simulink model "Instalatie_cu_filtru"  (R2024b)
settings: Solver=VariableStepAuto  StartTime=0.0  StopTime=1000  RelTol=1e-3  EnableMultiTasking=on
values from neighbouring files (symbols this model uses):
  k = 0.046    [Coeficienti.m]
  k11 = k2^2 + 4* (k - k3) * k1    (= 0.1165386)    [Coeficienti.m]
  k12 = 8* (k - k3)    (= 0.3728)    [Coeficienti.m]
  k13 = 2* (k - k3)    (= 0.0932)    [Coeficienti.m]
  k2 = -0.015    [Coeficienti.m]
  keta = 8e-5    (= 8e-05)    [Coeficienti.m]
  u0 = 6.6    [Coeficienti.m]
settings Model: Creator=otudo  LastModifiedBy=receaalex
settings SolverCC: AlgebraicLoopSolver=TrustRegion
settings DataIOCC: ReturnWorkspaceOutputs=off
settings OptimizationCC: LifeSpan=inf
settings DebuggingCC: UnconnectedInputMsg=warning  UnconnectedOutputMsg=warning  UnconnectedLineMsg=warning  SFUnexpectedBacktrackingDiag=warning  SFNoUnconditionalDefaultTransitionDiag=warning  ArithmeticOperatorsInVariantConditions=warning
settings ModelReferenceCC: EnableRefExpFcnMdlSchedulingChecks=on
settings SFSimCC: SimUseLocalCustomCode=off  CustomCodeUndefinedFunction=UseInterfaceOnly
settings RTWCC: RTWUseLocalCustomCode=off  GPUComputeCapability=3.5
settings CodeAppCC: StateflowObjectComments=on
settings GRTTargetCC: TargetLangStandard=C89/C90 (ANSI)
settings ConfigComp: CovMetricSettings=dw  CovSaveCumulativeToWorkspaceVar=on  CovSaveSingleToWorkspaceVar=on  CovExternalEMLEnable=off

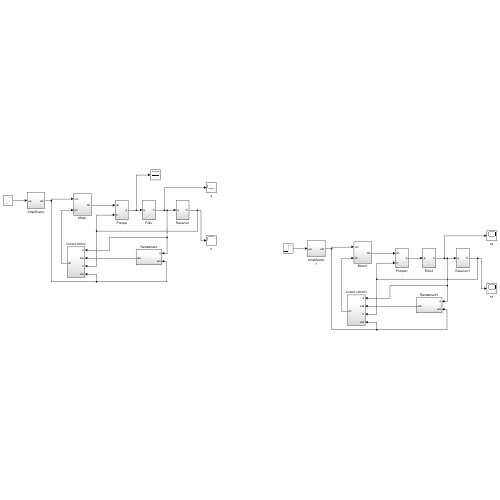
[thumbnail: Simulink's stored preview of the top-level diagram]
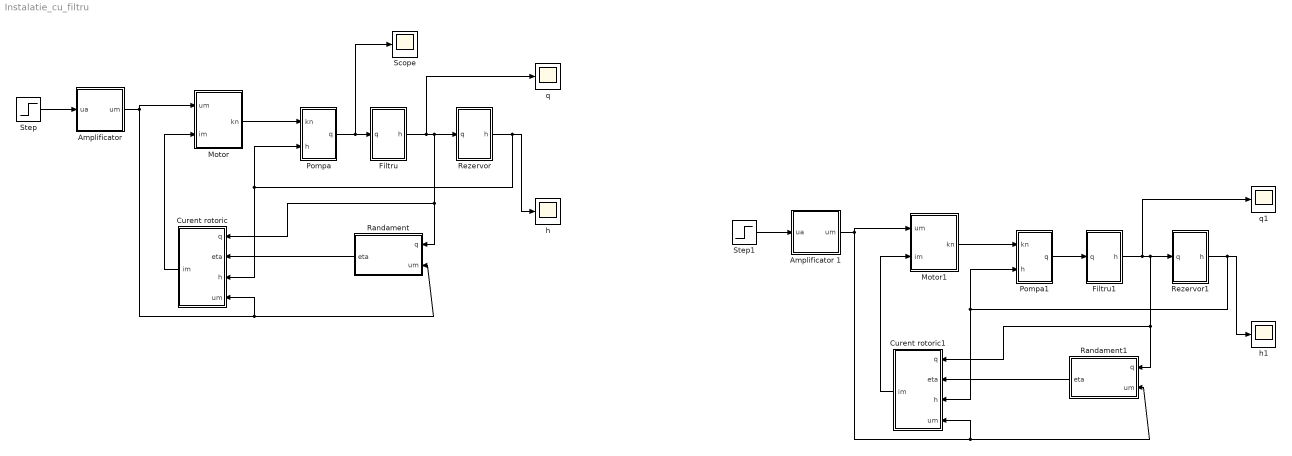
== system Instalatie_cu_filtru ==
  "Amplificator " : Subsystem
  Amplificator 1 : Subsystem
  Curent rotoric : Subsystem
  Curent rotoric1 : Subsystem
  Filtru : Subsystem
  Filtru1 : Subsystem
  Motor : Subsystem
  Motor1 : Subsystem
  Pompa : Subsystem
  Pompa1 : Subsystem
  Randament : Subsystem
  Randament1 : Subsystem
  Rezervor : Subsystem
  Rezervor1 : Subsystem
  Scope : Scope
  Step : Step  Before=u0  After=u0+0.5  SampleTime=0
  Step1 : Step  After=u0  SampleTime=0
  h : Scope
  h1 : Scope
  q : Scope
  q1 : Scope
  wires:
  Filtru/1(h) -> q/1, Curent rotoric/1(q), Randament/1(q), Rezervor/1(q)
  Step/1 -> "Amplificator "/1(ua)
  Randament/1(eta) -> Curent rotoric/2(eta)
  Rezervor/1(h) -> Curent rotoric/3(h), Pompa/2(h), h/1
  Pompa/1(q) -> Scope/1, Filtru/1(q)
  Curent rotoric/1(im) -> Motor/2(im)
  "Amplificator "/1(um) -> Curent rotoric/4(um), Randament/2(um), Motor/1(um)
  Motor/1(kn) -> Pompa/1(kn)
  Pompa1/1(q) -> Filtru1/1(q)
  Motor1/1(kn) -> Pompa1/1(kn)
  Step1/1 -> Amplificator 1/1(ua)
  Rezervor1/1(h) -> Curent rotoric1/3(h), Pompa1/2(h), h1/1
  Randament1/1(eta) -> Curent rotoric1/2(eta)
  Amplificator 1/1(um) -> Curent rotoric1/4(um), Randament1/2(um), Motor1/1(um)
  Curent rotoric1/1(im) -> Motor1/2(im)
  Filtru1/1(h) -> q1/1, Curent rotoric1/1(q), Randament1/1(q), Rezervor1/1(q)

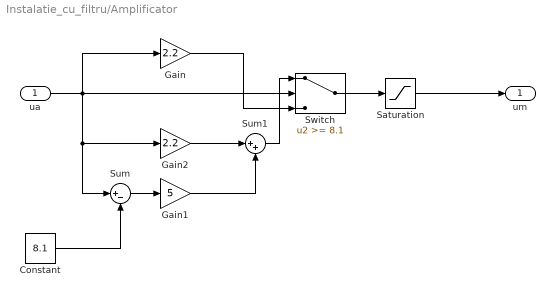
== system Instalatie_cu_filtru/Amplificator  ==
  ua : Inport
  Constant : Constant  Value=8.1
  Gain : Gain  Gain=2.2
  Gain1 : Gain  Gain=5
  Gain2 : Gain  Gain=2.2
  Saturation : Saturate  UpperLimit=22  LowerLimit=0
  Sum : Sum  Inputs=|+-
  Sum1 : Sum  Inputs=|++
  Switch : Switch  Threshold=8.1  SaturateOnIntegerOverflow=off  InputSameDT=off
  um : Outport
  wires:
  Gain/1 -> Switch/3
  Gain1/1 -> Sum1/2
  Switch/1 -> Saturation/1
  Constant/1 -> Sum/2
  Gain2/1 -> Sum1/1
  Sum/1 -> Gain1/1
  Saturation/1 -> um/1
  ua/1 -> Sum/1, Gain2/1, Gain/1, Switch/2
  Sum1/1 -> Switch/1

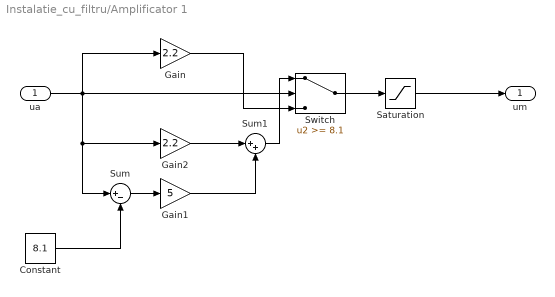
== system Instalatie_cu_filtru/Amplificator 1 ==
  ua : Inport
  Constant : Constant  Value=8.1
  Gain : Gain  Gain=2.2
  Gain1 : Gain  Gain=5
  Gain2 : Gain  Gain=2.2
  Saturation : Saturate  UpperLimit=22  LowerLimit=0
  Sum : Sum  Inputs=|+-
  Sum1 : Sum  Inputs=|++
  Switch : Switch  Threshold=8.1  SaturateOnIntegerOverflow=off  InputSameDT=off
  um : Outport
  wires:
  Gain/1 -> Switch/3
  Gain1/1 -> Sum1/2
  Switch/1 -> Saturation/1
  Constant/1 -> Sum/2
  Gain2/1 -> Sum1/1
  Sum/1 -> Gain1/1
  Saturation/1 -> um/1
  ua/1 -> Sum/1, Gain2/1, Gain/1, Switch/2
  Sum1/1 -> Switch/1

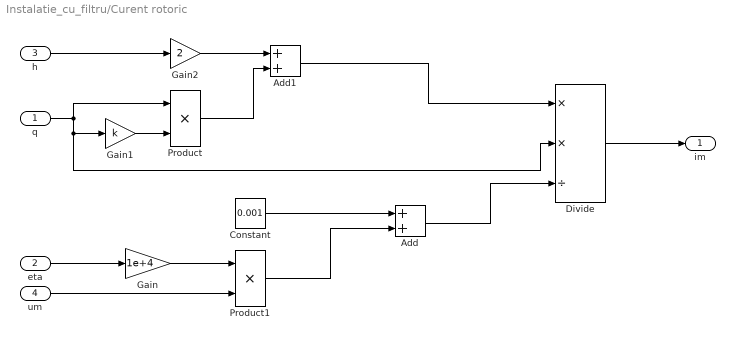
== system Instalatie_cu_filtru/Curent rotoric ==
  q : Inport
  eta : Inport  Port=2
  h : Inport  Port=3
  um : Inport  Port=4
  Add : Sum
  Add1 : Sum
  Constant : Constant  Value=0.001
  Divide : Product  Inputs=**/
  Gain : Gain  Gain=1e+4
  Gain1 : Gain  Gain=k
  Gain2 : Gain  Gain=2
  Product : Product
  Product1 : Product
  im : Outport
  wires:
  Add1/1 -> Divide/1
  Constant/1 -> Add/1
  Add/1 -> Divide/3
  Gain1/1 -> Product/2
  Product/1 -> Add1/2
  um/1 -> Product1/2
  Product1/1 -> Add/2
  Divide/1 -> im/1
  Gain/1 -> Product1/1
  Gain2/1 -> Add1/1
  eta/1 -> Gain/1
  q/1 -> Divide/2, Gain1/1, Product/1
  h/1 -> Gain2/1

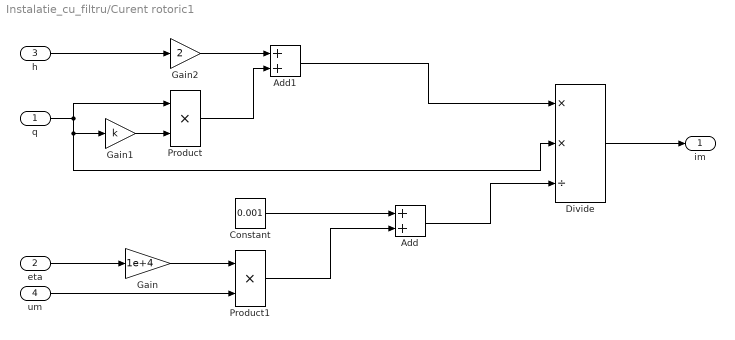
== system Instalatie_cu_filtru/Curent rotoric1 ==
  q : Inport
  eta : Inport  Port=2
  h : Inport  Port=3
  um : Inport  Port=4
  Add : Sum
  Add1 : Sum
  Constant : Constant  Value=0.001
  Divide : Product  Inputs=**/
  Gain : Gain  Gain=1e+4
  Gain1 : Gain  Gain=k
  Gain2 : Gain  Gain=2
  Product : Product
  Product1 : Product
  im : Outport
  wires:
  Add1/1 -> Divide/1
  Constant/1 -> Add/1
  Add/1 -> Divide/3
  Gain1/1 -> Product/2
  Product/1 -> Add1/2
  um/1 -> Product1/2
  Product1/1 -> Add/2
  Divide/1 -> im/1
  Gain/1 -> Product1/1
  Gain2/1 -> Add1/1
  eta/1 -> Gain/1
  q/1 -> Divide/2, Gain1/1, Product/1
  h/1 -> Gain2/1

== system Instalatie_cu_filtru/Filtru ==
  q : Inport
  Integrator : Integrator  InitialCondition=36.6
  Sum : Sum  Inputs=|+-
  h : Outport
  wires:
  Sum/1 -> Integrator/1
  q/1 -> Sum/1
  Integrator/1 -> h/1, Sum/2

== system Instalatie_cu_filtru/Filtru1 ==
  q : Inport
  Integrator : Integrator
  Sum : Sum  Inputs=|+-
  h : Outport
  wires:
  Sum/1 -> Integrator/1
  q/1 -> Sum/1
  Integrator/1 -> h/1, Sum/2

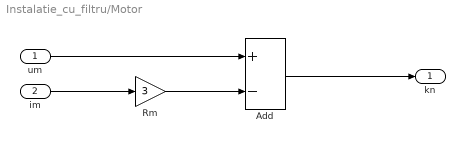
== system Instalatie_cu_filtru/Motor ==
  um : Inport
  im : Inport  Port=2
  Add : Sum  Inputs=+-
  "Rm " : Gain  Gain=3
  kn : Outport
  wires:
  "Rm "/1 -> Add/2
  Add/1 -> kn/1
  um/1 -> Add/1
  im/1 -> "Rm "/1

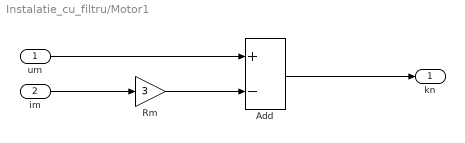
== system Instalatie_cu_filtru/Motor1 ==
  um : Inport
  im : Inport  Port=2
  Add : Sum  Inputs=+-
  "Rm " : Gain  Gain=3
  kn : Outport
  wires:
  "Rm "/1 -> Add/2
  Add/1 -> kn/1
  um/1 -> Add/1
  im/1 -> "Rm "/1

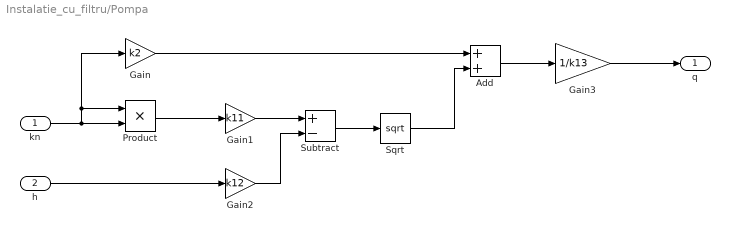
== system Instalatie_cu_filtru/Pompa ==
  kn : Inport
  h : Inport  Port=2
  Add : Sum
  Gain : Gain  Gain=k2
  Gain1 : Gain  Gain=k11
  Gain2 : Gain  Gain=k12
  Gain3 : Gain  Gain=1/k13
  Product : Product
  Sqrt : Sqrt
  Subtract : Sum  Inputs=+-
  q : Outport
  wires:
  Gain3/1 -> q/1
  Sqrt/1 -> Add/2
  Add/1 -> Gain3/1
  h/1 -> Gain2/1
  Gain2/1 -> Subtract/2
  Gain1/1 -> Subtract/1
  Subtract/1 -> Sqrt/1
  Product/1 -> Gain1/1
  Gain/1 -> Add/1
  kn/1 -> Gain/1, Product/1, Product/2

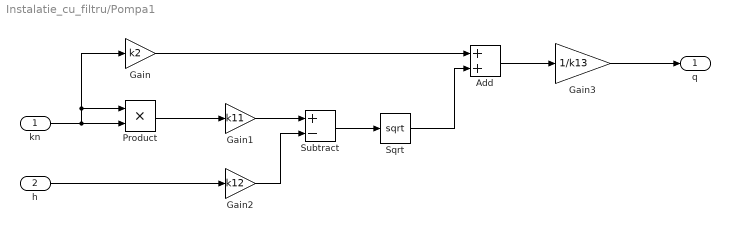
== system Instalatie_cu_filtru/Pompa1 ==
  kn : Inport
  h : Inport  Port=2
  Add : Sum
  Gain : Gain  Gain=k2
  Gain1 : Gain  Gain=k11
  Gain2 : Gain  Gain=k12
  Gain3 : Gain  Gain=1/k13
  Product : Product
  Sqrt : Sqrt
  Subtract : Sum  Inputs=+-
  q : Outport
  wires:
  Gain3/1 -> q/1
  Sqrt/1 -> Add/2
  Add/1 -> Gain3/1
  h/1 -> Gain2/1
  Gain2/1 -> Subtract/2
  Gain1/1 -> Subtract/1
  Subtract/1 -> Sqrt/1
  Product/1 -> Gain1/1
  Gain/1 -> Add/1
  kn/1 -> Gain/1, Product/1, Product/2

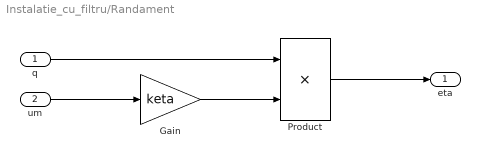
== system Instalatie_cu_filtru/Randament ==
  q : Inport
  um : Inport  Port=2
  Gain : Gain  Gain=keta
  Product : Product
  eta : Outport
  wires:
  Gain/1 -> Product/2
  Product/1 -> eta/1
  q/1 -> Product/1
  um/1 -> Gain/1

== system Instalatie_cu_filtru/Randament1 ==
  q : Inport
  um : Inport  Port=2
  Gain : Gain  Gain=keta
  Product : Product
  eta : Outport
  wires:
  Gain/1 -> Product/2
  Product/1 -> eta/1
  q/1 -> Product/1
  um/1 -> Gain/1

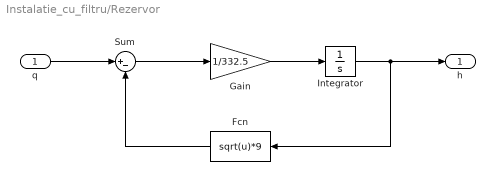
== system Instalatie_cu_filtru/Rezervor ==
  q : Inport
  Fcn : Fcn  Expr=sqrt(u)*9
  Gain : Gain  Gain=1/332.5
  Integrator : Integrator  InitialCondition=16.4
  Sum : Sum  Inputs=|+-
  h : Outport
  wires:
  q/1 -> Sum/1
  Sum/1 -> Gain/1
  Integrator/1 -> h/1, Fcn/1
  Fcn/1 -> Sum/2
  Gain/1 -> Integrator/1

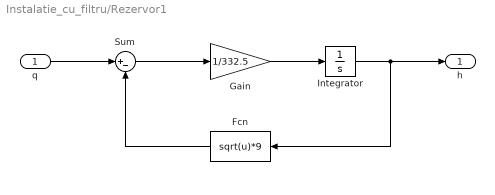
== system Instalatie_cu_filtru/Rezervor1 ==
  q : Inport
  Fcn : Fcn  Expr=sqrt(u)*9
  Gain : Gain  Gain=1/332.5
  Integrator : Integrator
  Sum : Sum  Inputs=|+-
  h : Outport
  wires:
  q/1 -> Sum/1
  Sum/1 -> Gain/1
  Integrator/1 -> h/1, Fcn/1
  Fcn/1 -> Sum/2
  Gain/1 -> Integrator/1
